simulink model "reaction_wheels_non_ideal_case"  (R2015b)
settings: Solver=FixedStepAuto  StartTime=0.0  StopTime=500  FixedStep=0.001  RelTol=1e-3
undefined symbols (not defined in the file): tau_w
settings Model: Creator=150010037  LastModifiedBy=150010037

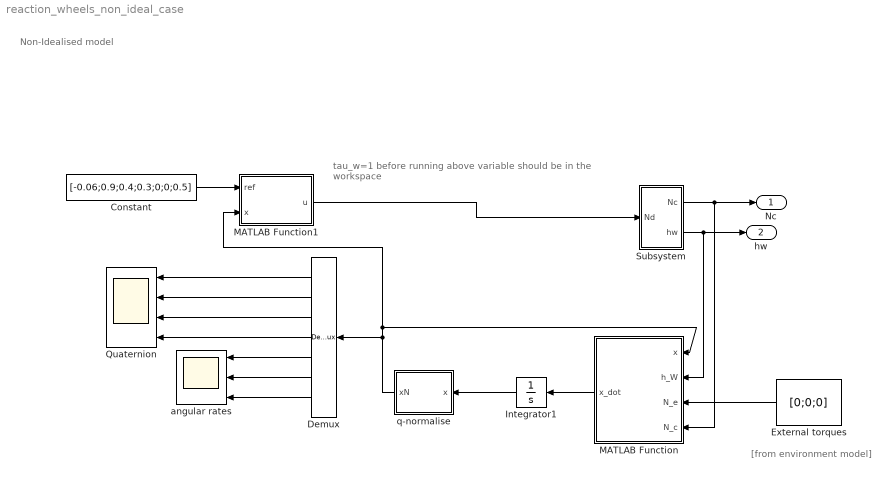
== system reaction_wheels_non_ideal_case ==
  note: tau_w=1
      | before running above variable should be in the workspace
  note: Non-Idealised model
  note: [from environment model]
  Constant : Constant  Value=[-0.06;0.9;0.4;0.3;0;0;0.5]
  Demux : Demux  Outputs=7
  "External torques " : Constant  Value=[0;0;0]
  Integrator1 : Integrator  InitialCondition=[2;3;5;3;3;2;6]
  MATLAB Function : MATLAB Function  TreatAsAtomicUnit=on
  MATLAB Function1 : MATLAB Function  TreatAsAtomicUnit=on
  Quaternion : Scope  NumInputPorts=4
  Subsystem : Subsystem
  angular rates : Scope  NumInputPorts=3
  q-normalise : MATLAB Function  TreatAsAtomicUnit=on
  Nc : Outport
  hw : Outport  Port=2
  wires:
  MATLAB Function/1(x_dot) -> Integrator1/1
  Integrator1/1 -> q-normalise/1(x)
  q-normalise/1(xN) -> MATLAB Function1/2(x), MATLAB Function/1(x), Demux/1
  "External torques "/1 -> MATLAB Function/3(N_e)
  Demux/4 -> Quaternion/4
  Demux/1 -> Quaternion/1
  Demux/2 -> Quaternion/2
  Demux/3 -> Quaternion/3
  Demux/7 -> angular rates/3
  Demux/6 -> angular rates/2
  Demux/5 -> angular rates/1
  Subsystem/2(hw) -> hw/1, MATLAB Function/2(h_W)
  Subsystem/1(Nc) -> Nc/1, MATLAB Function/4(N_c)
  Constant/1 -> MATLAB Function1/1(ref)
  MATLAB Function1/1(u) -> Subsystem/1(Nd)

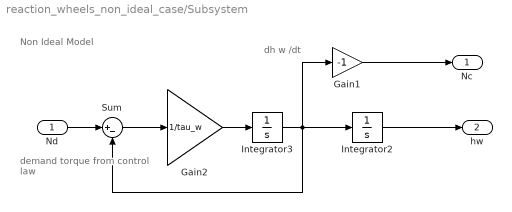
== system reaction_wheels_non_ideal_case/Subsystem ==
  note: Non Ideal Model
  note: dh w /dt
  note: demand torque
      | from control law
  Nd : Inport
  Gain1 : Gain  Gain=-1
  Gain2 : Gain  Gain=1/tau_w
  Integrator2 : Integrator
  Integrator3 : Integrator
  Sum : Sum  Inputs=|+-
  Nc : Outport
  hw : Outport  Port=2
  wires:
  Sum/1 -> Gain2/1
  Gain1/1 -> Nc/1
  Integrator3/1 -> Gain1/1, Integrator2/1, Sum/2
  Gain2/1 -> Integrator3/1
  Nd/1 -> Sum/1
  Integrator2/1 -> hw/1

== matlab function reaction_wheels_non_ideal_case/MATLAB Function1 ==
  data: ref input; x input; u output
function u = fcn(ref,x)
r=ref;
%quaternion error calculation
q_ref=[r(4) r(3) -r(2) -r(1) ;-r(3) r(4) r(1) r(2);r(2) -r(1) r(4) -r(3);r(1) r(2) r(3) r(4)];
q_s=x(1:4);
q_e=q_ref * q_s;
q1_e=[q_e(1)*q_e(4);q_e(2)*q_e(4);q_e(3)*q_e(4)];
%angular velocity error calculation
w_s=x(5:7);
w_r=r(5:7);
w_e=w_s -w_r;
kp=0.002; kpd =0.001;
u=-kp*q1_e - kpd*w_e;

== matlab function reaction_wheels_non_ideal_case/MATLAB Function ==
  data: x input; x_dot output; h_W input; N_e input; N_c input
function x_dot= fcn(x,h_W,N_e,N_c)
%W_dot calculation
w = x(5:7);
S_W=[ 0 -w(3) w(2);w(3) 0 w(1);-w(2) w(1) 0;];
I_s=[14.3 0 0;0 13.6 0; 0 0 4.6 ];

w_dot=-I_s\S_W*I_s*w - I_s\S_W*h_W + I_s\N_c + I_s\N_e;      %I_s\ means inv(I_s)*Ne

%q_dot calculation
q = x(1:4);
W = ...
    [ 0 w(3) -w(2) w(1);
      -w(3) 0 w(1) w(2);
      w(2) -w(1) 0 w(3);
      -w(1) -w(2) -w(3) 0];
  
q_dot = 0.5 * W * q;
x_dot=[q_dot;w_dot];

== matlab function reaction_wheels_non_ideal_case/q-normalise ==
  data: x input; xN output
function xN  = fcn(x)

q = x(1:4);
q = q/sqrt(dot(q,q));
xN = [q; x(5:7)];
